simulink model "fxpdemo_preconvert"  (Simulink 5.0)
settings: Solver=FixedStepDiscrete  SolverMode=SingleTasking  StartTime=0.0  StopTime=200.0  FixedStep=1  RelTol=1e-3
settings Model: RequirementInfo=9  MinMaxOverflowLogging=ForceOff  Creator=andyb  LastModifiedBy=andyb  ExtModeTrigMode=oneshot  ExtModeArmWhenConnect=off  ExtModeAutoUpdateStatusClock=off  LimitDataPoints=off  IntegerOverflowMsg=none  ParameterDowncastMsg=warning  ParameterOverflowMsg=warning  ParameterPrecisionLossMsg=none  BooleanDataType=off  RTWOptions="-aRollThreshold=5 -aShowEliminatedStatements=1 -aRTWVerbose=1 -aLocalBlockOutputs=1 -aInlineInvariantSignals=1 -aLogVarNameModifier=\"rt_\" -aExtMode=0"

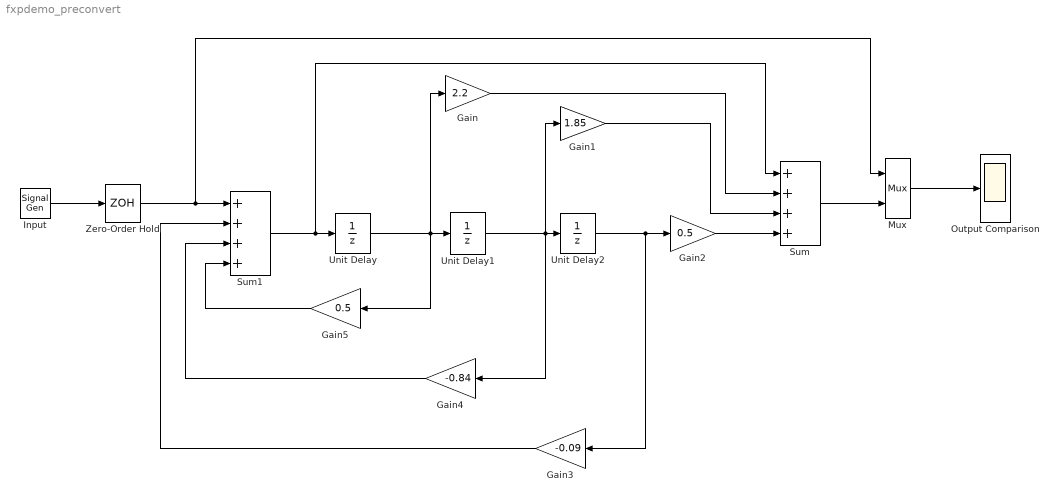
== system fxpdemo_preconvert ==
  Gain : Gain  Gain=2.2  SaturateOnIntegerOverflow=on
  Gain1 : Gain  Gain=1.85  SaturateOnIntegerOverflow=on
  Gain2 : Gain  Gain=0.5  SaturateOnIntegerOverflow=on
  Gain3 : Gain  Orientation=left  Gain=-0.09  SaturateOnIntegerOverflow=on
  Gain4 : Gain  Orientation=left  Gain=-0.84  SaturateOnIntegerOverflow=on
  Gain5 : Gain  Orientation=left  Gain=0.5  SaturateOnIntegerOverflow=on
  Input : SignalGenerator  WaveForm=square  Frequency=0.005
  Mux : Mux  Inputs=2
  Output Comparison : Scope
      settings: TickLabels=on  TimeRange=200  YMin=-8  YMax=10  SaveName=OutputComparison
  Sum : Sum  Inputs=4  SaturateOnIntegerOverflow=on  InputSameDT=on
  Sum1 : Sum  Inputs=4  SaturateOnIntegerOverflow=on  InputSameDT=on
  Unit Delay : UnitDelay
  Unit Delay1 : UnitDelay
  Unit Delay2 : UnitDelay
  Zero-Order Hold : ZeroOrderHold
  wires:
  Input/1 -> Zero-Order Hold/1
  Sum1/1 -> Unit Delay/1, Sum/1
  Gain5/1 -> Sum1/4
  Unit Delay/1 -> Unit Delay1/1, Gain5/1, Gain/1
  Gain4/1 -> Sum1/3
  Unit Delay1/1 -> Unit Delay2/1, Gain4/1, Gain1/1
  Gain3/1 -> Sum1/2
  Gain2/1 -> Sum/4
  Gain1/1 -> Sum/3
  Gain/1 -> Sum/2
  Unit Delay2/1 -> Gain2/1, Gain3/1
  Zero-Order Hold/1 -> Sum1/1, Mux/1
  Sum/1 -> Mux/2
  Mux/1 -> Output Comparison/1
